simulink model "New_enth2temp"  (Simulink 7.6)
settings: Solver=FixedStepDiscrete  StartTime=0.0  StopTime=10  FixedStep=1  RelTol=1e-3
libraries: lib_Enthalpy2Temperature x1
settings Model: Creator=awohlfei  LastModifiedBy=drhf
settings DebuggingCC: FcnCallInpInsideContextMsg=Enable All
settings GRTTargetCC: CombineOutputUpdateFcns=on

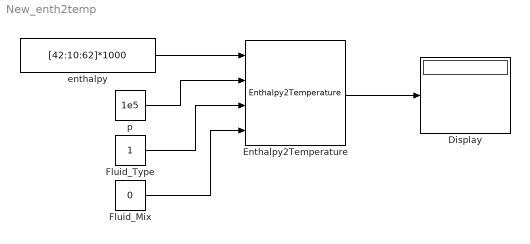
== system New_enth2temp ==
  Display : Display
  Enthalpy2Temperature : lib_Enthalpy2Temperature/Enthalpy2Temperature  SystemSampleTime=-1  VariantObject=CarlibClassic  DEBUGLEVEL=WARNINGLEVEL  MAXTOTALMESSAGES=inf  MAXCONSECUTIVEMESSAGES=inf  WRITETOFILE=0  FILENAME='errors.txt'
  Fluid_Mix : Constant  Value=0
  Fluid_Type : Constant
  enthalpy : Constant  Value=[42:10:62]*1000
  p : Constant  Value=1e5
  wires:
  enthalpy/1 -> Enthalpy2Temperature/1
  Enthalpy2Temperature/1 -> Display/1
  p/1 -> Enthalpy2Temperature/2
  Fluid_Type/1 -> Enthalpy2Temperature/3
  Fluid_Mix/1 -> Enthalpy2Temperature/4
